simulink model "otu19"  (R2018a)
settings: Solver=ode45  StartTime=0.0  StopTime=5  RelTol=1e-3  EnableMultiTasking=on
settings Model: Creator=bukova.2018  LastModifiedBy=kincharov.2018
settings DataIOCC: LimitDataPoints=on  SaveFormat=Array  SignalLoggingSaveFormat=ModelDataLogs
settings OptimizationCC: ExpressionDepthLimit=2147483647  LifeSpan=inf
settings DebuggingCC: UnderspecifiedInitializationDetection=Classic  MergeDetectMultiDrivingBlocksExec=none  SolverPrmCheckMsg=warning  FcnCallInpInsideContextMsg=warning  StateNameClashWarn=warning  SFUnexpectedBacktrackingDiag=warning  SFNoUnconditionalDefaultTransitionDiag=warning  SFExecutionAtInitializationDiag=none
settings HardwareCC: ProdBitPerPointer=32  ProdBitPerSizeT=32  ProdBitPerPtrDiffT=32  ProdLargestAtomicFloat=None  ProdIntDivRoundTo=Undefined  ProdEndianess=Unspecified  ProdWordSize=32  ProdHWDeviceType=32-bit Generic
settings ModelReferenceCC: PropagateSignalLabelsOutOfModel=off
settings CodeAppCC: StateflowObjectComments=on
settings GRTTargetCC: TargetLangStandard=C89/C90 (ANSI)  GeneratePreprocessorConditionals=Disable all  CombineOutputUpdateFcns=off  GRTInterface=on
settings ConfigComp: CovMetricSettings=dw  CovHtmlReporting=on  CovSaveCumulativeToWorkspaceVar=on  CovSaveSingleToWorkspaceVar=on  CovExternalEMLEnable=off

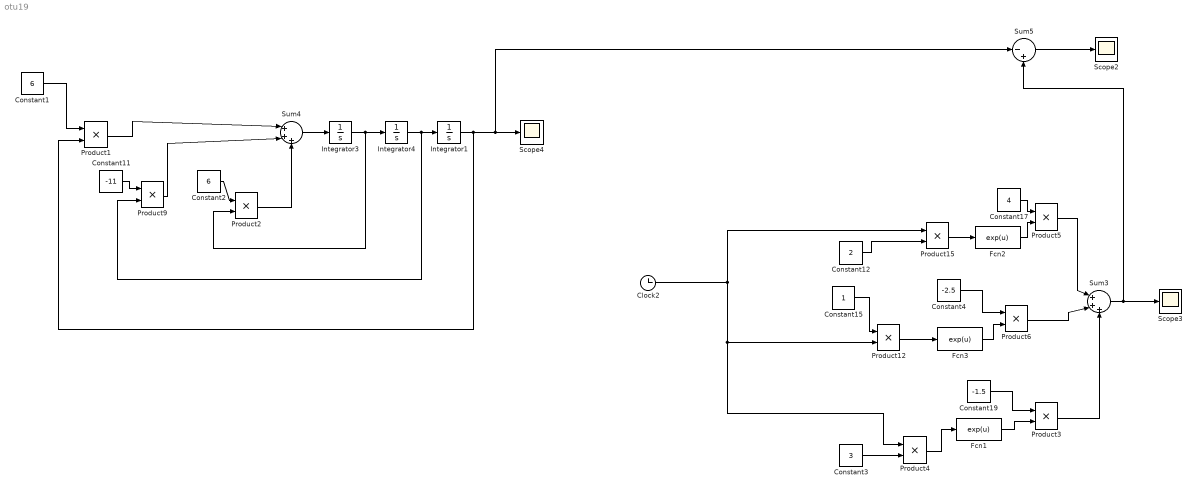
== system otu19 ==
  Clock2 : Clock
  Constant1 : Constant  Value=6
  Constant11 : Constant  Value=-11
  Constant12 : Constant  Value=2
  Constant15 : Constant
  Constant17 : Constant  Value=4
  Constant19 : Constant  Value=-1.5
  Constant2 : Constant  Value=6
  Constant3 : Constant  Value=3
  Constant4 : Constant  Value=-2.5
  Fcn1 : Fcn  Expr=exp(u)
  Fcn2 : Fcn  Expr=exp(u)
  Fcn3 : Fcn  Expr=exp(u)
  Integrator1 : Integrator
  Integrator3 : Integrator
  Integrator4 : Integrator  InitialCondition=1
  Product{1..6,9,12,15} (9 alike) : Product  RndMeth=Zero
  Scope2 : Scope
  Scope3 : Scope
  Scope4 : Scope
  Sum3 : Sum  Inputs=|+++
  Sum4 : Sum  Inputs=|+++
  Sum5 : Sum  Inputs=|-+
  wires:
  Product5/1 -> Sum3/1
  Constant11/1 -> Product9/1
  Constant15/1 -> Product12/1
  Constant12/1 -> Product15/2
  Constant17/1 -> Product5/1
  Fcn2/1 -> Product5/2
  Product15/1 -> Fcn2/1
  Sum5/1 -> Scope2/1
  Clock2/1 -> Product4/1, Product12/2, Product15/1
  Sum3/1 -> Scope3/1, Sum5/2
  Product9/1 -> Sum4/2
  Integrator4/1 -> Product9/2, Integrator1/1
  Constant1/1 -> Product1/1
  Product1/1 -> Sum4/1
  Sum4/1 -> Integrator3/1
  Constant2/1 -> Product2/1
  Product2/1 -> Sum4/3
  Integrator1/1 -> Product1/2, Sum5/1, Scope4/1
  Integrator3/1 -> Product2/2, Integrator4/1
  Constant19/1 -> Product3/1
  Fcn1/1 -> Product3/2
  Product3/1 -> Sum3/3
  Constant3/1 -> Product4/2
  Product4/1 -> Fcn1/1
  Product12/1 -> Fcn3/1
  Constant4/1 -> Product6/1
  Fcn3/1 -> Product6/2
  Product6/1 -> Sum3/2
